simulink library "momentum_flight_control_v1"  (R2022a)
settings: Solver=VariableStepAuto  StartTime=0.0  StopTime=10.0  RelTol=1e-3
undefined symbols (not defined in the file): biasVectorConstraint_feet, Config, ConstraintMatrix_feet, DiscIntNeverNeededParam, Frames
libraries: WBToolboxLibrary x40
(part 1 of 2)
settings Model: Creator=gnava  LastModifiedBy=gnava
settings SolverCC: AlgebraicLoopSolver=TrustRegion
settings DebuggingCC: UnconnectedInputMsg=warning  UnconnectedOutputMsg=warning  UnconnectedLineMsg=warning  SFMachineParentedDataDiag=warning
settings RTWCC: DLArmComputeVersion=19.05

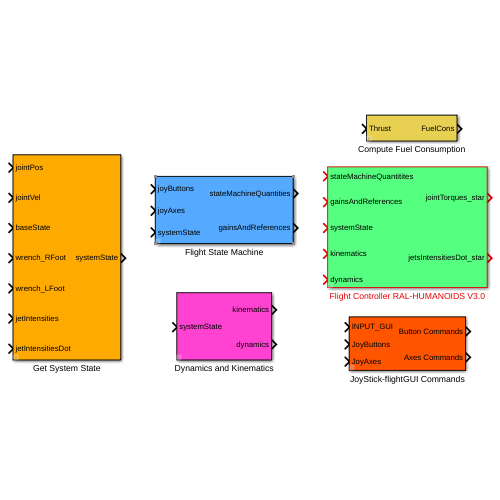
[thumbnail: Simulink's stored preview of the top-level diagram]
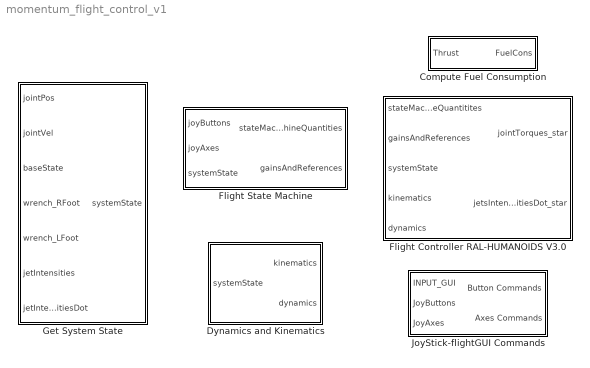
== system momentum_flight_control_v1 ==
  Compute Fuel Consumption : Subsystem  mask{Parameter1=Config}
      mask prompts: Parameter1 "Specify the parameters struct"
      mask DialogControl DescGroupVar Prompt: Compute Fuel Consumption
      mask DialogControl DescTextVar Prompt: Calculates the fuel consumption while flying.
  Dynamics and Kinematics : Subsystem  mask{Parameter1=Config, Parameter2=Frames}
      mask prompts: Parameter1 "Specify the parameters struct"; Parameter2 "Specify the frame names struct"
      mask DialogControl DescGroupVar Prompt: Dynamics and Kinematics
      mask DialogControl DescTextVar Prompt: Computes the dynamics and kinematics quantities that are required by the iRonCub flight controller.
  Flight Controller RAL-HUMANOIDS V3.0 : Subsystem  mask{Parameter1=Config}
      mask prompts: Parameter1 "Specify the parameters struct"
      mask DialogControl DescGroupVar Prompt: Flight Controller RAL-HUMANOIDS
      mask DialogControl DescTextVar Prompt: This block implements the momentum-based flight controller decribed in RAL 2018 and HUMANOIDS 2018 papers.
      mask DialogControl Control3 Prompt: References:
      mask DialogControl Control5 Prompt: RAL 2018 paper
      mask DialogControl Control5 Callback: web https://ieeexplore.ieee.org/document/7997895
      mask DialogControl Control6 Prompt: HUMANOIDS 2018 paper
      mask DialogControl Control6 Callback: web https://ieeexplore.ieee.org/document/8624985
  Flight State Machine : Subsystem  mask{Parameter1=Config, Parameter2=Frames}
      mask prompts: Parameter1 "Specify the parameters struct"; Parameter2 "Specify the frame names struct"
      mask DialogControl DescGroupVar Prompt: Flight State Machine
      mask DialogControl DescTextVar Prompt: Implements a state machine that allows iRonCub to take off, fly, and land. It also allows the user to provide reference trajectories to the robot via joypad or a control GUI.
  Get System State : Subsystem  mask{Parameter1=Frames}
      mask prompts: Parameter1 "Specify the frame names struct"
      mask DialogControl DescGroupVar Prompt: Get System State
      mask DialogControl DescTextVar Prompt: Computes the iRonCub state vector while flying.
      mask DialogControl DescGroupVar_copy Prompt: Parameters
  JoyStick-flightGUI Commands : Subsystem  mask{Parameter1=Config}
      mask prompts: Parameter1 "Specify the parameters struct"
      mask DialogControl DescGroupVar Prompt: Joystick/flightGUI Commands
      mask DialogControl DescTextVar Prompt: Generates commands for the flight state machine. Commands are provided by the user either using a joypad or with the native GUI.

== system momentum_flight_control_v1/Compute Fuel Consumption ==
  Thrust : Inport
  Discrete-Time Integrator : DiscreteIntegrator  SampleTime=Config.tStep  ICPrevOutput=DiscIntNeverNeededParam  ICPrevScaledInput=DiscIntNeverNeededParam
  Get the Current Fuel Consumption : MATLAB Function  TreatAsAtomicUnit=on
  FuelCons : Outport
  wires:
  Thrust/1 -> Get the Current Fuel Consumption/1(thrusts)
  Get the Current Fuel Consumption/1(fuelConsCurr) -> Discrete-Time Integrator/1
  Discrete-Time Integrator/1 -> FuelCons/1

== system momentum_flight_control_v1/Dynamics and Kinematics ==
  systemState : Inport
  Bus Creator1 : BusCreator  Inputs=5
  Bus Creator2 : BusCreator  Inputs=12
  Bus Selector : BusSelector  OutputSignals=w_H_b,jointPos,w_baseTwist,jointVel
  Dynamic Quantities : Subsystem
  Kinematic Quantities : Subsystem
  kinematics : Outport  VectorParamsAs1DForOutWhenUnconnected=off
  dynamics : Outport  Port=2  VectorParamsAs1DForOutWhenUnconnected=off
  wires:
  systemState/1 -> Bus Selector/1
  Bus Selector/1 -> Dynamic Quantities/2(w_H_b), Kinematic Quantities/1(w_H_b)  "<w_H_b>"
  Bus Selector/2 -> Dynamic Quantities/3(jointPos), Kinematic Quantities/2(jointPos)  "<jointPos>"
  Bus Selector/3 -> Dynamic Quantities/4(w_baseTwist), Kinematic Quantities/3(w_baseTwist)  "<w_baseTwist>"
  Bus Selector/4 -> Dynamic Quantities/5(jointVel), Kinematic Quantities/4(jointVel)  "<jointVel>"
  Dynamic Quantities/4(CMM) -> Bus Creator1/4  "CMM"
  Dynamic Quantities/3(L) -> Bus Creator1/3  "L"
  Dynamic Quantities/2("h ") -> Bus Creator1/2  "h"
  Dynamic Quantities/1(M) -> Bus Creator1/1  "M"
  Bus Creator1/1 -> dynamics/1
  Bus Creator2/1 -> kinematics/1
  Kinematic Quantities/1(J_jets) -> Bus Creator2/1  "J_jets"
  Kinematic Quantities/2(J_CoM) -> Bus Creator2/2  "J_CoM"
  Kinematic Quantities/3(w_R_b) -> Bus Creator2/3  "w_R_b"
  Kinematic Quantities/4(J_LFoot) -> Bus Creator2/4  "J_LFoot"
  Kinematic Quantities/5(J_RFoot) -> Bus Creator2/5  "J_RFoot"
  Kinematic Quantities/6(JDot_LFoot_nu) -> Bus Creator2/6  "JDot_LFoot_nu"
  Kinematic Quantities/7(JDot_RFoot_nu) -> Bus Creator2/7  "JDot_RFoot_nu"
  Kinematic Quantities/8(w_H_LFoot) -> Bus Creator2/8  "w_H_LFoot"
  Kinematic Quantities/9(w_H_RFoot) -> Bus Creator2/9  "w_H_RFoot"
  Kinematic Quantities/10(matrixOfJetsAxes) -> Bus Creator2/10  "matrixOfJetAxes"
  Kinematic Quantities/11(matrixOfJetsArms) -> Bus Creator2/11  "matrixOfJetsArms"
  Kinematic Quantities/12(posCoM) -> Bus Creator2/12, Dynamic Quantities/1(posCoM)  "posCoM"
  Dynamic Quantities/5(w_I_c) -> Bus Creator1/5  "w_I_c"

== system momentum_flight_control_v1/Flight Controller RAL-HUMANOIDS V3.0 ==
  stateMachineQuantitites : Inport
  gainsAndReferences : Inport  Port=2
  systemState : Inport  Port=3
  kinematics : Inport  Port=4
  dynamics : Inport  Port=5
  Joint Torque Control for Flying : Subsystem
  Momentum Control for Flying : Subsystem
  jointTorques_star : Outport  VectorParamsAs1DForOutWhenUnconnected=off
  jetsIntensitiesDot_star : Outport  Port=2  VectorParamsAs1DForOutWhenUnconnected=off
  wires:
  stateMachineQuantitites/1 -> Joint Torque Control for Flying/3(stateMachineQuantitites), Momentum Control for Flying/1(stateMachineQuantitites)
  gainsAndReferences/1 -> Joint Torque Control for Flying/4(gainsAndReferences), Momentum Control for Flying/2(gainsAndReferences)
  systemState/1 -> Joint Torque Control for Flying/5(systemState), Momentum Control for Flying/3(systemState)
  kinematics/1 -> Joint Torque Control for Flying/6(kinematics), Momentum Control for Flying/4(kinematics)
  dynamics/1 -> Joint Torque Control for Flying/7(dynamics), Momentum Control for Flying/5(dynamics)
  Momentum Control for Flying/2(contactForces_star) -> Joint Torque Control for Flying/2(contactForces_star)
  Joint Torque Control for Flying/1(jointTorques_star) -> jointTorques_star/1
  Momentum Control for Flying/3(jetsIntensitiesDot_star) -> jetsIntensitiesDot_star/1
  Momentum Control for Flying/1(jointVel_star) -> Joint Torque Control for Flying/1(jointVel_star)

== system momentum_flight_control_v1/Flight State Machine ==
  joyButtons : Inport
  joyAxes : Inport  Port=2
  systemState : Inport  Port=3
  Bus Selector : BusSelector  OutputSignals=jointPos
  Compute Gains And References : Subsystem
  Take Off/Landing State Detector : Subsystem
  stateMachineQuantities : Outport  VectorParamsAs1DForOutWhenUnconnected=off
  gainsAndReferences : Outport  Port=2  VectorParamsAs1DForOutWhenUnconnected=off
  wires:
  systemState/1 -> Take Off/Landing State Detector/1(systemState), Compute Gains And References/3(systemState), Bus Selector/1
  joyButtons/1 -> Take Off/Landing State Detector/2(joyButtons), Compute Gains And References/2(joyButtons)
  joyAxes/1 -> Compute Gains And References/1(joyAxes)
  Compute Gains And References/1(gainsAndReferences) -> gainsAndReferences/1
  Bus Selector/1 -> Compute Gains And References/4(jointPos)  "<jointPos>"
  Take Off/Landing State Detector/1(stateMachineQuantities) -> stateMachineQuantities/1, Compute Gains And References/5(stateMachineQuantities)

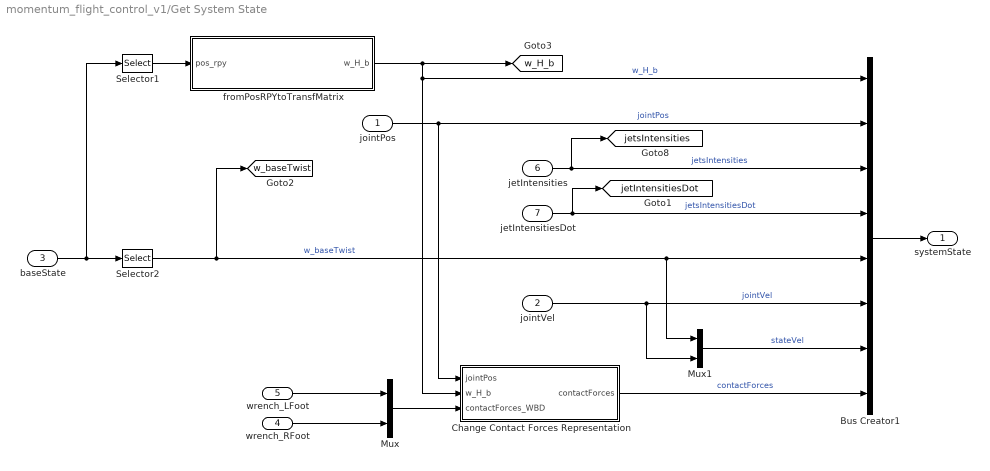
== system momentum_flight_control_v1/Get System State ==
  jointPos : Inport
  jointVel : Inport  Port=2
  baseState : Inport  Port=3
  wrench_RFoot : Inport  Port=4
  wrench_LFoot : Inport  Port=5
  jetIntensities : Inport  Port=6
  jetIntensitiesDot : Inport  Port=7
  Bus Creator1 : BusCreator  Inputs=8
  Change Contact Forces Representation : Subsystem
  Mux : Mux  Inputs=2
  Mux1 : Mux  Inputs=2
  Selector1 : Selector  InputPortWidth=18  IndexOptions=Index vector (dialog)  Indices=[1:6]  OutputSizes=1
  Selector2 : Selector  InputPortWidth=18  IndexOptions=Index vector (dialog)  Indices=[7:12]  OutputSizes=1
  fromPosRPYtoTransfMatrix : MATLAB Function  TreatAsAtomicUnit=on
  systemState : Outport  VectorParamsAs1DForOutWhenUnconnected=off
  tag scope: jetIntensitiesDot=global, jetsIntensities=global, w_H_b=global, w_baseTwist=global
  wires:
  fromPosRPYtoTransfMatrix/1(w_H_b) -> [w_H_b], Change Contact Forces Representation/2(w_H_b), Bus Creator1/1  "w_H_b"
  Mux1/1 -> Bus Creator1/7  "stateVel"
  jetIntensitiesDot/1 -> [jetIntensitiesDot], Bus Creator1/4  "jetsIntensitiesDot"
  wrench_RFoot/1 -> Mux/2
  Mux/1 -> Change Contact Forces Representation/3(contactForces_WBD)
  jointPos/1 -> Change Contact Forces Representation/1(jointPos), Bus Creator1/2  "jointPos"
  jetIntensities/1 -> Bus Creator1/3, [jetsIntensities]  "jetsIntensities"
  Bus Creator1/1 -> systemState/1
  wrench_LFoot/1 -> Mux/1
  Selector1/1 -> fromPosRPYtoTransfMatrix/1(pos_rpy)
  jointVel/1 -> Mux1/2, Bus Creator1/6  "jointVel"
  baseState/1 -> Selector1/1, Selector2/1
  Selector2/1 -> [w_baseTwist], Mux1/1, Bus Creator1/5  "w_baseTwist"
  Change Contact Forces Representation/1(contactForces) -> Bus Creator1/8  "contactForces"

== system momentum_flight_control_v1/JoyStick-flightGUI Commands ==
  INPUT_GUI : Inport
  JoyButtons : Inport  Port=2
  JoyAxes : Inport  Port=3
  Constant : Constant  Value=Config.USE_NATIVE_GUI
  Replace Joystick with Native GUI : MATLAB Function  TreatAsAtomicUnit=on
  Switch1 : Switch  Criteria=u2 > Threshold  SaturateOnIntegerOverflow=off  InputSameDT=off
  Switch2 : Switch  Criteria=u2 > Threshold  SaturateOnIntegerOverflow=off  InputSameDT=off
  Button Commands : Outport  VectorParamsAs1DForOutWhenUnconnected=off
  Axes Commands : Outport  Port=2  VectorParamsAs1DForOutWhenUnconnected=off
  wires:
  INPUT_GUI/1 -> Replace Joystick with Native GUI/1(gui_input)
  Switch1/1 -> Button Commands/1
  Switch2/1 -> Axes Commands/1
  Constant/1 -> Switch2/2, Switch1/2
  JoyButtons/1 -> Switch1/3
  JoyAxes/1 -> Switch2/3
  Replace Joystick with Native GUI/2(joyAxes) -> Switch2/1
  Replace Joystick with Native GUI/1(joyButtons) -> Switch1/1

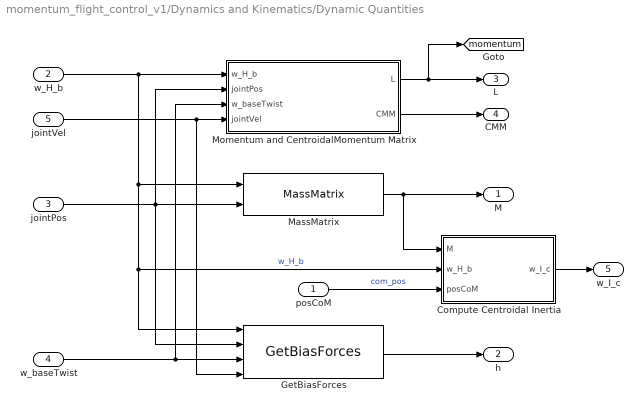
== system momentum_flight_control_v1/Dynamics and Kinematics/Dynamic Quantities ==
  posCoM : Inport
  w_H_b : Inport  Port=2
  jointPos : Inport  Port=3
  w_baseTwist : Inport  Port=4
  jointVel : Inport  Port=5
  Compute Centroidal Inertia : Subsystem
  GetBiasForces : WBToolboxLibrary/Model/Dynamics/GetBiasForces
      settings: SourceProductName=WholeBodyToolbox
  MassMatrix : WBToolboxLibrary/Model/Dynamics/MassMatrix
      settings: SourceProductName=WholeBodyToolbox
  Momentum and CentroidalMomentum Matrix : Subsystem
  M : Outport  VectorParamsAs1DForOutWhenUnconnected=off
  "h " : Outport  Port=2  VectorParamsAs1DForOutWhenUnconnected=off
  L : Outport  Port=3  VectorParamsAs1DForOutWhenUnconnected=off
  CMM : Outport  Port=4  VectorParamsAs1DForOutWhenUnconnected=off
  w_I_c : Outport  Port=5  VectorParamsAs1DForOutWhenUnconnected=off
  tag scope: momentum=global
  wires:
  w_H_b/1 -> Momentum and CentroidalMomentum Matrix/1(w_H_b), GetBiasForces/1, Compute Centroidal Inertia/2(w_H_b), MassMatrix/1  "w_H_b"
  w_baseTwist/1 -> Momentum and CentroidalMomentum Matrix/3(w_baseTwist), GetBiasForces/3
  jointVel/1 -> Momentum and CentroidalMomentum Matrix/4(jointVel), GetBiasForces/4
  MassMatrix/1 -> Compute Centroidal Inertia/1(M), M/1
  GetBiasForces/1 -> "h "/1
  Momentum and CentroidalMomentum Matrix/2(CMM) -> CMM/1
  Momentum and CentroidalMomentum Matrix/1(L) -> L/1, [momentum]
  jointPos/1 -> GetBiasForces/2, MassMatrix/2, Momentum and CentroidalMomentum Matrix/2(jointPos)
  Compute Centroidal Inertia/1(w_I_c) -> w_I_c/1
  posCoM/1 -> Compute Centroidal Inertia/3(posCoM)  "com_pos"

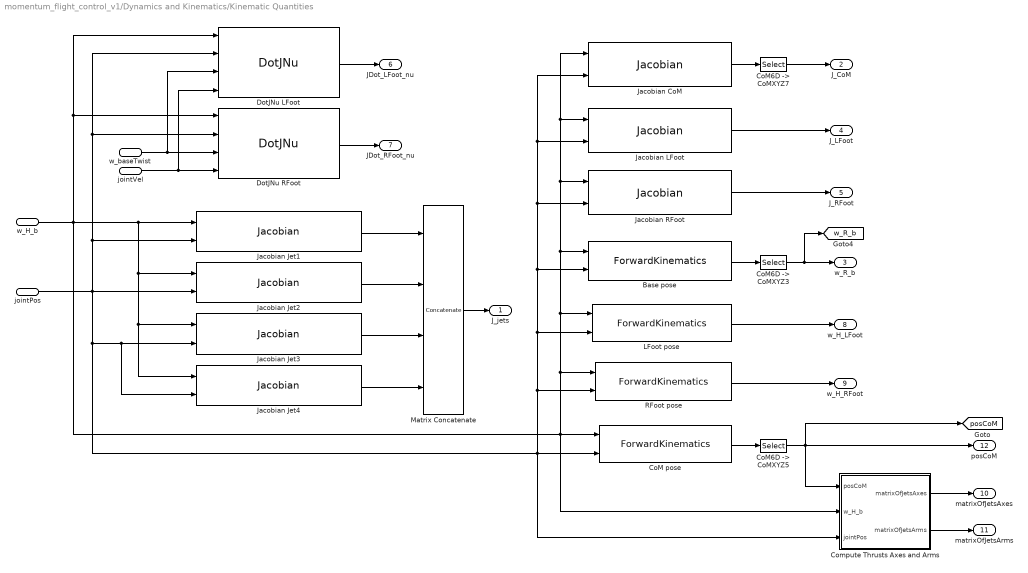
== system momentum_flight_control_v1/Dynamics and Kinematics/Kinematic Quantities ==
  w_H_b : Inport
  jointPos : Inport  Port=2
  w_baseTwist : Inport  Port=3
  jointVel : Inport  Port=4
  Base pose : WBToolboxLibrary/Model/Kinematics/ForwardKinematics  frameName=Frames.BASE_LINK
      settings: SourceProductName=WholeBodyToolbox
  CoM pose : WBToolboxLibrary/Model/Kinematics/ForwardKinematics  frameName=Frames.COM_FRAME
      settings: SourceProductName=WholeBodyToolbox
  "CoM6D -> CoMXYZ3" : Selector  NumberOfDimensions=2  InputPortWidth=7  IndexOptions=Index vector (dialog),Index vector (dialog)  Indices=[1 2 3],[1 2 3]  OutputSizes=1,1
  "CoM6D -> CoMXYZ5" : Selector  NumberOfDimensions=2  InputPortWidth=7  IndexOptions=Index vector (dialog),Index vector (dialog)  Indices=[1 2 3],[4]  OutputSizes=1,1
  "CoM6D -> CoMXYZ7" : Selector  NumberOfDimensions=2  InputPortWidth=7  IndexOptions=Index vector (dialog),Index vector (dialog)  Indices=[1 2 3],[1:6+Config.N_DOF]  OutputSizes=1,1
  Compute Thrusts Axes and Arms : Subsystem
  DotJNu LFoot : WBToolboxLibrary/Model/Jacobians/DotJNu  frameName=Frames.LFOOT_FRAME
      settings: SourceProductName=WholeBodyToolbox
  DotJNu RFoot : WBToolboxLibrary/Model/Jacobians/DotJNu  frameName=Frames.RFOOT_FRAME
      settings: SourceProductName=WholeBodyToolbox
  Jacobian CoM : WBToolboxLibrary/Model/Jacobians/Jacobian  frameName=Frames.COM_FRAME
      settings: SourceProductName=WholeBodyToolbox
  Jacobian Jet1 : WBToolboxLibrary/Model/Jacobians/Jacobian  frameName=Frames.JET1_FRAME
      settings: SourceProductName=WholeBodyToolbox
  Jacobian Jet2 : WBToolboxLibrary/Model/Jacobians/Jacobian  frameName=Frames.JET2_FRAME
      settings: SourceProductName=WholeBodyToolbox
  Jacobian Jet3 : WBToolboxLibrary/Model/Jacobians/Jacobian  frameName=Frames.JET3_FRAME
      settings: SourceProductName=WholeBodyToolbox
  Jacobian Jet4 : WBToolboxLibrary/Model/Jacobians/Jacobian  frameName=Frames.JET4_FRAME
      settings: SourceProductName=WholeBodyToolbox
  Jacobian LFoot : WBToolboxLibrary/Model/Jacobians/Jacobian  frameName=Frames.LFOOT_FRAME
      settings: SourceProductName=WholeBodyToolbox
  Jacobian RFoot : WBToolboxLibrary/Model/Jacobians/Jacobian  frameName=Frames.RFOOT_FRAME
      settings: SourceProductName=WholeBodyToolbox
  LFoot pose : WBToolboxLibrary/Model/Kinematics/ForwardKinematics  frameName=Frames.LFOOT_FRAME
      settings: SourceProductName=WholeBodyToolbox
  Matrix Concatenate : Concatenate  NumInputs=4  Mode=Multidimensional array
  RFoot pose : WBToolboxLibrary/Model/Kinematics/ForwardKinematics  frameName=Frames.RFOOT_FRAME
      settings: SourceProductName=WholeBodyToolbox
  J_jets : Outport  VectorParamsAs1DForOutWhenUnconnected=off
  J_CoM : Outport  Port=2  VectorParamsAs1DForOutWhenUnconnected=off
  w_R_b : Outport  Port=3  VectorParamsAs1DForOutWhenUnconnected=off
  J_LFoot : Outport  Port=4  VectorParamsAs1DForOutWhenUnconnected=off
  J_RFoot : Outport  Port=5  VectorParamsAs1DForOutWhenUnconnected=off
  JDot_LFoot_nu : Outport  Port=6  VectorParamsAs1DForOutWhenUnconnected=off
  JDot_RFoot_nu : Outport  Port=7  VectorParamsAs1DForOutWhenUnconnected=off
  w_H_LFoot : Outport  Port=8  VectorParamsAs1DForOutWhenUnconnected=off
  w_H_RFoot : Outport  Port=9  VectorParamsAs1DForOutWhenUnconnected=off
  matrixOfJetsAxes : Outport  Port=10  VectorParamsAs1DForOutWhenUnconnected=off
  matrixOfJetsArms : Outport  Port=11  VectorParamsAs1DForOutWhenUnconnected=off
  posCoM : Outport  Port=12  VectorParamsAs1DForOutWhenUnconnected=off
  tag scope: posCoM=global, w_R_b=global
  wires:
  Matrix Concatenate/1 -> J_jets/1
  CoM pose/1 -> "CoM6D -> CoMXYZ5"/1
  "CoM6D -> CoMXYZ5"/1 -> posCoM/1, [posCoM], Compute Thrusts Axes and Arms/1(posCoM)
  w_H_b/1 -> LFoot pose/1, Base pose/1, Jacobian LFoot/1, Jacobian CoM/1, Jacobian RFoot/1, RFoot pose/1, CoM pose/1, Compute Thrusts Axes and Arms/2(w_H_b), DotJNu LFoot/1, DotJNu RFoot/1, Jacobian Jet4/1, Jacobian Jet3/1, Jacobian Jet2/1, Jacobian Jet1/1
  "CoM6D -> CoMXYZ3"/1 -> w_R_b/1, [w_R_b]
  jointPos/1 -> Jacobian Jet4/2, Jacobian Jet3/2, Compute Thrusts Axes and Arms/3(jointPos), LFoot pose/2, Jacobian RFoot/2, Jacobian LFoot/2, Jacobian CoM/2, Base pose/2, RFoot pose/2, CoM pose/2, Jacobian Jet2/2, DotJNu LFoot/2, DotJNu RFoot/2, Jacobian Jet1/2
  Jacobian CoM/1 -> "CoM6D -> CoMXYZ7"/1
  Jacobian RFoot/1 -> J_RFoot/1
  Jacobian LFoot/1 -> J_LFoot/1
  DotJNu RFoot/1 -> JDot_RFoot_nu/1
  DotJNu LFoot/1 -> JDot_LFoot_nu/1
  jointVel/1 -> DotJNu RFoot/4, DotJNu LFoot/4
  w_baseTwist/1 -> DotJNu LFoot/3, DotJNu RFoot/3
  RFoot pose/1 -> w_H_RFoot/1
  LFoot pose/1 -> w_H_LFoot/1
  Base pose/1 -> "CoM6D -> CoMXYZ3"/1
  Compute Thrusts Axes and Arms/2(matrixOfJetsArms) -> matrixOfJetsArms/1
  Compute Thrusts Axes and Arms/1(matrixOfJetsAxes) -> matrixOfJetsAxes/1
  Jacobian Jet1/1 -> Matrix Concatenate/1
  Jacobian Jet2/1 -> Matrix Concatenate/2
  Jacobian Jet3/1 -> Matrix Concatenate/3
  Jacobian Jet4/1 -> Matrix Concatenate/4
  "CoM6D -> CoMXYZ7"/1 -> J_CoM/1

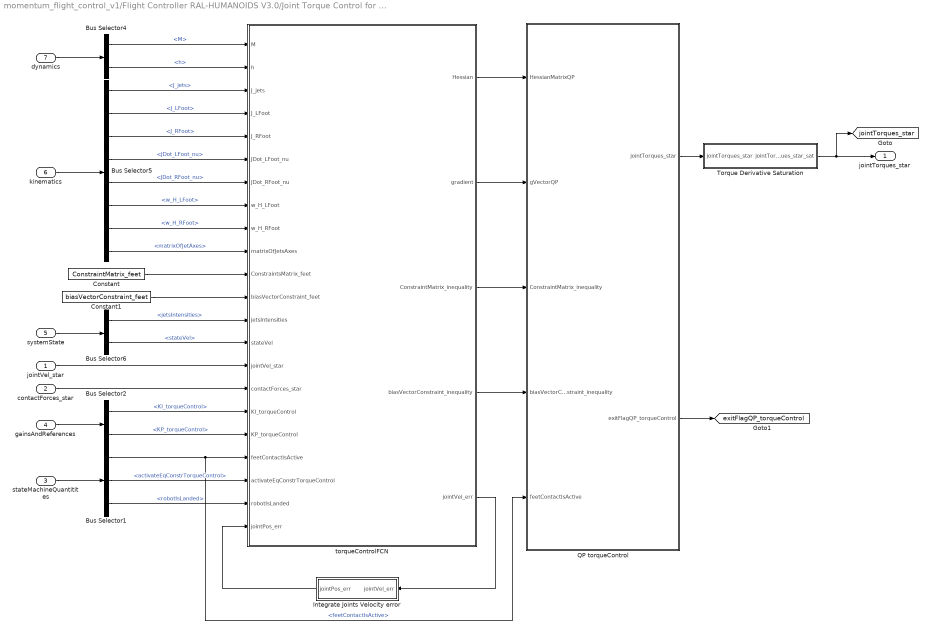
== system momentum_flight_control_v1/Flight Controller RAL-HUMANOIDS V3.0/Joint Torque Control for Flying ==
  jointVel_star : Inport
  contactForces_star : Inport  Port=2
  stateMachineQuantitites : Inport  Port=3
  gainsAndReferences : Inport  Port=4
  systemState : Inport  Port=5
  kinematics : Inport  Port=6
  dynamics : Inport  Port=7
  Bus Selector1 : BusSelector  OutputSignals=feetContactIsActive,activateEqConstrTorqueControl,robotIsLanded
  Bus Selector2 : BusSelector  OutputSignals=KI_torqueControl,KP_torqueControl
  Bus Selector4 : BusSelector  OutputSignals=M,h
  Bus Selector5 : BusSelector  OutputSignals=J_jets,J_LFoot,J_RFoot,JDot_LFoot_nu,JDot_RFoot_nu,w_H_LFoot,w_H_RFoot,matrixOfJetAxes
  Bus Selector6 : BusSelector  OutputSignals=jetsIntensities,stateVel
  Constant : Constant  Value=ConstraintMatrix_feet
  Constant1 : Constant  Value=biasVectorConstraint_feet
  Integrate Joints Velocity error : Subsystem
  QP torqueControl : Subsystem
  Torque Derivative Saturation : Subsystem
  torqueControlFCN : MATLAB Function  TreatAsAtomicUnit=on
  jointTorques_star : Outport  VectorParamsAs1DForOutWhenUnconnected=off
  tag scope: exitFlagQP_torqueControl=global, jointTorques_star=global
  wires:
  Bus Selector6/2 -> torqueControlFCN/14(stateVel)  "<stateVel>"
  dynamics/1 -> Bus Selector4/1
  systemState/1 -> Bus Selector6/1
  kinematics/1 -> Bus Selector5/1
  Bus Selector4/1 -> torqueControlFCN/1(M)  "<M>"
  Bus Selector4/2 -> torqueControlFCN/2(h)  "<h>"
  Bus Selector5/1 -> torqueControlFCN/3(J_jets)  "<J_jets>"
  Bus Selector5/2 -> torqueControlFCN/4(J_LFoot)  "<J_LFoot>"
  Bus Selector5/3 -> torqueControlFCN/5(J_RFoot)  "<J_RFoot>"
  Bus Selector5/4 -> torqueControlFCN/6(JDot_LFoot_nu)  "<JDot_LFoot_nu>"
  Bus Selector5/5 -> torqueControlFCN/7(JDot_RFoot_nu)  "<JDot_RFoot_nu>"
  Bus Selector5/6 -> torqueControlFCN/8(w_H_LFoot)  "<w_H_LFoot>"
  Bus Selector5/7 -> torqueControlFCN/9(w_H_RFoot)  "<w_H_RFoot>"
  Constant1/1 -> torqueControlFCN/12(biasVectorConstraint_feet)
  Constant/1 -> torqueControlFCN/11(ConstraintsMatrix_feet)
  contactForces_star/1 -> torqueControlFCN/16(contactForces_star)
  QP torqueControl/1(jointTorques_star) -> Torque Derivative Saturation/1(jointTorques_star)
  QP torqueControl/2(exitFlagQP_torqueControl) -> [exitFlagQP_torqueControl]
  Bus Selector6/1 -> torqueControlFCN/13(jetsIntensities)  "<jetsIntensities>"
  stateMachineQuantitites/1 -> Bus Selector1/1
  Bus Selector1/1 -> QP torqueControl/5(feetContactIsActive), torqueControlFCN/19(feetContactIsActive)  "<feetContactIsActive>"
  gainsAndReferences/1 -> Bus Selector2/1
  Bus Selector2/1 -> torqueControlFCN/17(KI_torqueControl)  "<KI_torqueControl>"
  Bus Selector2/2 -> torqueControlFCN/18(KP_torqueControl)  "<KP_torqueControl>"
  torqueControlFCN/1(Hessian) -> QP torqueControl/1(HessianMatrixQP)
  torqueControlFCN/2(gradient) -> QP torqueControl/2(gVectorQP)
  torqueControlFCN/3(ConstraintMatrix_inequality) -> QP torqueControl/3(ConstraintMatrix_inequality)
  torqueControlFCN/4(biasVectorConstraint_inequality) -> QP torqueControl/4(biasVectorConstraint_inequality)
  jointVel_star/1 -> torqueControlFCN/15(jointVel_star)
  Bus Selector5/8 -> torqueControlFCN/10(matrixOfJetsAxes)  "<matrixOfJetAxes>"
  Integrate Joints Velocity error/1(jointPos_err) -> torqueControlFCN/22(jointPos_err)
  torqueControlFCN/5(jointVel_err) -> Integrate Joints Velocity error/1(jointVel_err)
  Bus Selector1/3 -> torqueControlFCN/21(robotIsLanded)  "<robotIsLanded>"
  Bus Selector1/2 -> torqueControlFCN/20(activateEqConstrTorqueControl)  "<activateEqConstrTorqueControl>"
  Torque Derivative Saturation/1(jointTorques_star_sat) -> [jointTorques_star], jointTorques_star/1

== system momentum_flight_control_v1/Flight Controller RAL-HUMANOIDS V3.0/Momentum Control for Flying ==
  stateMachineQuantitites : Inport
  gainsAndReferences : Inport  Port=2
  systemState : Inport  Port=3
  kinematics : Inport  Port=4
  dynamics : Inport  Port=5
  Momentum Control : Subsystem
  QP Solver and Integrate Contact Forces Derivative : Subsystem
  jointVel_star : Outport  VectorParamsAs1DForOutWhenUnconnected=off
  contactForces_star : Outport  Port=2  VectorParamsAs1DForOutWhenUnconnected=off
  jetsIntensitiesDot_star : Outport  Port=3  VectorParamsAs1DForOutWhenUnconnected=off
  wires:
  kinematics/1 -> Momentum Control/3(kinematics)
  dynamics/1 -> Momentum Control/4(dynamics)
  gainsAndReferences/1 -> Momentum Control/5(gainsAndReferences)
  stateMachineQuantitites/1 -> Momentum Control/6(stateMachineQuantitites), QP Solver and Integrate Contact Forces Derivative/5(stateMachineQuantities)
  Momentum Control/1(HessianMatrixQP) -> QP Solver and Integrate Contact Forces Derivative/1(HessianMatrixQP)
  Momentum Control/2(gVectorQP) -> QP Solver and Integrate Contact Forces Derivative/2(gVectorQP)
  Momentum Control/3(lowerBoundQP) -> QP Solver and Integrate Contact Forces Derivative/3(lowerBoundQP)
  Momentum Control/4(uppeBoundQP) -> QP Solver and Integrate Contact Forces Derivative/4(upperBoundQP)
  QP Solver and Integrate Contact Forces Derivative/2(jetsIntensitiesDot_star) -> jetsIntensitiesDot_star/1
  QP Solver and Integrate Contact Forces Derivative/1(contactForces_star) -> Momentum Control/1(contactForces_hat), contactForces_star/1  "WARNING! estimated contact forces are assumed to be coincident with contactForces_star"
  QP Solver and Integrate Contact Forces Derivative/3(jointVel_star) -> jointVel_star/1
  systemState/1 -> Momentum Control/2(systemState), QP Solver and Integrate Contact Forces Derivative/6(systemState)

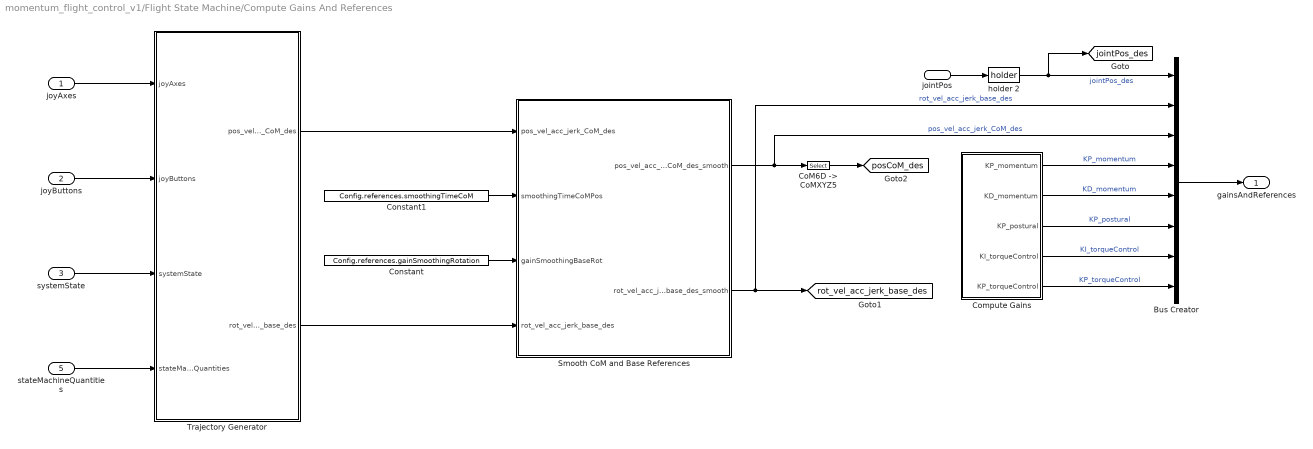
== system momentum_flight_control_v1/Flight State Machine/Compute Gains And References ==
  joyAxes : Inport
  joyButtons : Inport  Port=2
  systemState : Inport  Port=3
  jointPos : Inport  Port=4
  stateMachineQuantities : Inport  Port=5
  Bus Creator : BusCreator  Inputs=8
  "CoM6D -> CoMXYZ5" : Selector  NumberOfDimensions=2  InputPortWidth=7  IndexOptions=Index vector (dialog),Index vector (dialog)  Indices=[1 2 3],[1]  OutputSizes=1,1
  Compute Gains : Subsystem
  Constant : Constant  Value=Config.references.gainSmoothingRotation
  Constant1 : Constant  Value=Config.references.smoothingTimeCoM
  Smooth CoM and Base References : Subsystem
  Trajectory Generator : Subsystem
  holder 2 : WBToolboxLibrary/Utilities/holder 
      settings: SourceProductName=WholeBodyToolbox
  gainsAndReferences : Outport  VectorParamsAs1DForOutWhenUnconnected=off
  tag scope: jointPos_des=global, posCoM_des=global, rot_vel_acc_jerk_base_des=global
  wires:
  "CoM6D -> CoMXYZ5"/1 -> [posCoM_des]
  Smooth CoM and Base References/1(pos_vel_acc_jerk_CoM_des_smooth) -> "CoM6D -> CoMXYZ5"/1, Bus Creator/3  "pos_vel_acc_jerk_CoM_des"
  Constant1/1 -> Smooth CoM and Base References/2(smoothingTimeCoMPos)
  Smooth CoM and Base References/2(rot_vel_acc_jerk_base_des_smooth) -> [rot_vel_acc_jerk_base_des], Bus Creator/2  "rot_vel_acc_jerk_base_des"
  Compute Gains/5(KP_torqueControl) -> Bus Creator/8  "KP_torqueControl"
  Compute Gains/2(KD_momentum) -> Bus Creator/5  "KD_momentum"
  Compute Gains/1(KP_momentum) -> Bus Creator/4  "KP_momentum"
  Compute Gains/3(KP_postural) -> Bus Creator/6  "KP_postural"
  Constant/1 -> Smooth CoM and Base References/3(gainSmoothingBaseRot)
  Bus Creator/1 -> gainsAndReferences/1
  Compute Gains/4(KI_torqueControl) -> Bus Creator/7  "KI_torqueControl"
  holder 2/1 -> Bus Creator/1, [jointPos_des]  "jointPos_des"
  jointPos/1 -> holder 2/1
  joyAxes/1 -> Trajectory Generator/1(joyAxes)
  joyButtons/1 -> Trajectory Generator/2(joyButtons)
  systemState/1 -> Trajectory Generator/3(systemState)
  stateMachineQuantities/1 -> Trajectory Generator/4(stateMachineQuantities)
  Trajectory Generator/1(pos_vel_acc_jerk_CoM_des) -> Smooth CoM and Base References/1(pos_vel_acc_jerk_CoM_des)
  Trajectory Generator/2(rot_vel_acc_jerk_base_des) -> Smooth CoM and Base References/4(rot_vel_acc_jerk_base_des)

== system momentum_flight_control_v1/Flight State Machine/Take Off//Landing State Detector ==
  systemState : Inport
  joyButtons : Inport  Port=2
  Bus Creator : BusCreator  Inputs=6
  Bus Selector : BusSelector  OutputSignals=contactForces
  Demux : Demux  Outputs=[6;6]
  MATLAB Function : MATLAB Function  TreatAsAtomicUnit=on
  Vertical Forces Control : MATLAB Function  TreatAsAtomicUnit=on
  stateMachineQuantities : Outport  VectorParamsAs1DForOutWhenUnconnected=off
  tag scope: stateMachineQuantities=global
  wires:
  Vertical Forces Control/1(decreaseMaxFootVerticalForce) -> Bus Creator/1  "decreaseMaxFootVerticalForce"
  Vertical Forces Control/2(increaseMinFootVerticalForce) -> Bus Creator/2  "increaseMinFootVerticalForce"
  Bus Creator/1 -> [stateMachineQuantities], stateMachineQuantities/1
  systemState/1 -> Bus Selector/1
  joyButtons/1 -> Vertical Forces Control/1(joyButtons)
  Demux/2 -> MATLAB Function/2(wrench_r)
  Demux/1 -> MATLAB Function/1(wrench_l)
  Bus Selector/1 -> Demux/1  "<contactForces>"
  MATLAB Function/1(feetContactIsActive) -> Bus Creator/4  "feetContactIsActive"
  MATLAB Function/2(robotIsLanded) -> Bus Creator/5  "robotIsLanded"
  MATLAB Function/3(oneFootIsInContact) -> Bus Creator/6  "oneFootIsInContact"
  Vertical Forces Control/3(activateEqConstrTorqueControl) -> Bus Creator/3  "activateEqConstrTorqueControl"

== system momentum_flight_control_v1/Get System State/Change Contact Forces Representation ==
  jointPos : Inport
  w_H_b : Inport  Port=2
  contactForces_WBD : Inport  Port=3
  Change Contact Forces Representation : MATLAB Function  TreatAsAtomicUnit=on
  "CoM6D -> CoMXYZ1" : Selector  NumberOfDimensions=2  InputPortWidth=7  IndexOptions=Index vector (dialog),Index vector (dialog)  Indices=[1 2 3],[1 2 3]  OutputSizes=1,1
  "CoM6D -> CoMXYZ3" : Selector  NumberOfDimensions=2  InputPortWidth=7  IndexOptions=Index vector (dialog),Index vector (dialog)  Indices=[1 2 3],[1 2 3]  OutputSizes=1,1
  LFoot Pose : WBToolboxLibrary/Model/Kinematics/ForwardKinematics  frameName=Frames.LFOOT_FRAME
      settings: SourceProductName=WholeBodyToolbox
  Mux : Mux  Inputs=2
  RFoot Pose : WBToolboxLibrary/Model/Kinematics/ForwardKinematics  frameName=Frames.RFOOT_FRAME
      settings: SourceProductName=WholeBodyToolbox
  contactForces : Outport  VectorParamsAs1DForOutWhenUnconnected=off
  tag scope: wrench_LFoot=global, wrench_RFoot=global
  wires:
  Mux/1 -> contactForces/1
  Change Contact Forces Representation/2(mixed_f_r_sole) -> Mux/2, [wrench_RFoot]
  Change Contact Forces Representation/1(mixed_f_l_sole) -> Mux/1, [wrench_LFoot]
  jointPos/1 -> RFoot Pose/2, LFoot Pose/2
  w_H_b/1 -> RFoot Pose/1, LFoot Pose/1
  "CoM6D -> CoMXYZ1"/1 -> Change Contact Forces Representation/2(w_R_l_sole)
  LFoot Pose/1 -> "CoM6D -> CoMXYZ1"/1
  "CoM6D -> CoMXYZ3"/1 -> Change Contact Forces Representation/3(w_R_r_sole)
  RFoot Pose/1 -> "CoM6D -> CoMXYZ3"/1
  contactForces_WBD/1 -> Change Contact Forces Representation/1(contactForces_WBD)

== system momentum_flight_control_v1/Dynamics and Kinematics/Dynamic Quantities/Compute Centroidal Inertia ==
  M : Inport
  w_H_b : Inport  Port=2
  posCoM : Inport  Port=3
  Compute Centroidal Inertia : MATLAB Function  TreatAsAtomicUnit=on
  Selector : Selector  NumberOfDimensions=2  InputPortWidth=3  IndexOptions=Index vector (dialog),Index vector (dialog)  Indices=[1 2 3],4  OutputSizes=1,1
  w_I_c : Outport  VectorParamsAs1DForOutWhenUnconnected=off
  wires:
  M/1 -> Compute Centroidal Inertia/1(M)
  w_H_b/1 -> Selector/1
  Selector/1 -> Compute Centroidal Inertia/3(posBase)
  posCoM/1 -> Compute Centroidal Inertia/2(posCoM)
  Compute Centroidal Inertia/1(w_I_c) -> w_I_c/1

== system momentum_flight_control_v1/Dynamics and Kinematics/Dynamic Quantities/Momentum and CentroidalMomentum Matrix ==
  w_H_b : Inport
  jointPos : Inport  Port=2
  w_baseTwist : Inport  Port=3
  jointVel : Inport  Port=4
  CentroidalMomentum : WBToolboxLibrary/Model/Dynamics/CentroidalMomentum
      settings: SourceProductName=WholeBodyToolbox
  CentroidalTotalMomentumMatrix : WBToolboxLibrary/Model/Jacobians/CentroidalTotalMomentumMatrix
      settings: SourceProductName=WholeBodyToolbox
  L : Outport  VectorParamsAs1DForOutWhenUnconnected=off
  CMM : Outport  Port=2  VectorParamsAs1DForOutWhenUnconnected=off
  wires:
  w_baseTwist/1 -> CentroidalMomentum/3
  CentroidalMomentum/1 -> L/1
  w_H_b/1 -> CentroidalTotalMomentumMatrix/1, CentroidalMomentum/1
  jointPos/1 -> CentroidalTotalMomentumMatrix/2, CentroidalMomentum/2
  jointVel/1 -> CentroidalMomentum/4
  CentroidalTotalMomentumMatrix/1 -> CMM/1

== system momentum_flight_control_v1/Dynamics and Kinematics/Kinematic Quantities/Compute Thrusts Axes and Arms ==
  posCoM : Inport
  w_H_b : Inport  Port=2
  jointPos : Inport  Port=3
  Pose Jet 1 : WBToolboxLibrary/Model/Kinematics/ForwardKinematics  frameName=Frames.JET1_FRAME
      settings: SourceProductName=WholeBodyToolbox
  Pose Jet 2 : WBToolboxLibrary/Model/Kinematics/ForwardKinematics  frameName=Frames.JET2_FRAME
      settings: SourceProductName=WholeBodyToolbox
  Pose Jet 3 : WBToolboxLibrary/Model/Kinematics/ForwardKinematics  frameName=Frames.JET3_FRAME
      settings: SourceProductName=WholeBodyToolbox
  Pose Jet 4 : WBToolboxLibrary/Model/Kinematics/ForwardKinematics  frameName=Frames.JET4_FRAME
      settings: SourceProductName=WholeBodyToolbox
  Thrust Axes and Arms : MATLAB Function  TreatAsAtomicUnit=on
  matrixOfJetsAxes : Outport  VectorParamsAs1DForOutWhenUnconnected=off
  matrixOfJetsArms : Outport  Port=2  VectorParamsAs1DForOutWhenUnconnected=off
  wires:
  Pose Jet 2/1 -> Thrust Axes and Arms/2(w_H_J2)
  jointPos/1 -> Pose Jet 1/2, Pose Jet 2/2, Pose Jet 3/2, Pose Jet 4/2
  Pose Jet 1/1 -> Thrust Axes and Arms/1(w_H_J1)
  Pose Jet 3/1 -> Thrust Axes and Arms/3(w_H_J3)
  Pose Jet 4/1 -> Thrust Axes and Arms/4(w_H_J4)
  Thrust Axes and Arms/1(matrixOfJetsAxes) -> matrixOfJetsAxes/1
  Thrust Axes and Arms/2(matrixOfJetsArms) -> matrixOfJetsArms/1
  w_H_b/1 -> Pose Jet 4/1, Pose Jet 3/1, Pose Jet 2/1, Pose Jet 1/1
  posCoM/1 -> Thrust Axes and Arms/5(posCoM)

== system momentum_flight_control_v1/Flight Controller RAL-HUMANOIDS V3.0/Joint Torque Control for Flying/Integrate Joints Velocity error ==
  jointVel_err : Inport
  Constant : Constant  Value=zeros(Config.N_DOF,1)
  Discrete-Time Integrator1 : DiscreteIntegrator  InitialConditionSource=external  InitialCondition=zeros(Config.N_DOF,1)  SampleTime=Config.tStep  ICPrevOutput=DiscIntNeverNeededParam  ICPrevScaledInput=DiscIntNeverNeededParam
  jointPos_err : Outport  VectorParamsAs1DForOutWhenUnconnected=off
  tag scope: jointPos_err_integral=global
  wires:
  Discrete-Time Integrator1/1 -> jointPos_err/1, [jointPos_err_integral]
  jointVel_err/1 -> Discrete-Time Integrator1/1
  Constant/1 -> Discrete-Time Integrator1/2

== system momentum_flight_control_v1/Flight Controller RAL-HUMANOIDS V3.0/Joint Torque Control for Flying/QP torqueControl ==
  HessianMatrixQP : Inport
  gVectorQP : Inport  Port=2
  ConstraintMatrix_inequality : Inport  Port=3
  biasVectorConstraint_inequality : Inport  Port=4
  feetContactIsActive : Inport  Port=5
  Constant2 : Constant  Value=Config.sat.jointTorquesSaturation
  NOT : Logic  Operator=NOT  IconShape=distinctive  AllPortsSameDT=off  OutDataTypeStr=boolean
  Process QP Inputs Torque Control : MATLAB Function  TreatAsAtomicUnit=on
  QP torqueControl - balancing : Subsystem  TreatAsAtomicUnit=on
  QP torqueControl - flight : Subsystem  TreatAsAtomicUnit=on
  Select QP torqueControl Output : Subsystem
  jointTorques_star : Outport  VectorParamsAs1DForOutWhenUnconnected=off
  exitFlagQP_torqueControl : Outport  Port=2  VectorParamsAs1DForOutWhenUnconnected=off
  wires:
  feetContactIsActive/1 -> Select QP torqueControl Output/3(feetContactIsActive), QP torqueControl - balancing/Enable, NOT/1
  NOT/1 -> QP torqueControl - flight/Enable
  biasVectorConstraint_inequality/1 -> Process QP Inputs Torque Control/4(biasVectorInequalityConstr)
  ConstraintMatrix_inequality/1 -> Process QP Inputs Torque Control/3(InequalityConstrMatrix)
  HessianMatrixQP/1 -> Process QP Inputs Torque Control/1(HessianMatrixQP)
  gVectorQP/1 -> Process QP Inputs Torque Control/2(gVectorQP)
  Constant2/1 -> Process QP Inputs Torque Control/5(jointTorquesSaturation)
  Process QP Inputs Torque Control/8(H_flight) -> QP torqueControl - flight/1(H)
  Process QP Inputs Torque Control/9(g_flight) -> QP torqueControl - flight/2(g)
  Process QP Inputs Torque Control/10(ub_flight) -> QP torqueControl - flight/3(ub)
  Process QP Inputs Torque Control/11(lb_flight) -> QP torqueControl - flight/4(lb)
  Process QP Inputs Torque Control/7(ubEq_balancing) -> QP torqueControl - balancing/7(ubEq)
  Process QP Inputs Torque Control/6(lbEq_balancing) -> QP torqueControl - balancing/6(lbEq)
  Process QP Inputs Torque Control/5(Aeq_balancing) -> QP torqueControl - balancing/5(AEq)
  Process QP Inputs Torque Control/4(lb_balancing) -> QP torqueControl - balancing/4(lb)
  Process QP Inputs Torque Control/3(ub_balancing) -> QP torqueControl - balancing/3(ub)
  Process QP Inputs Torque Control/2(g_balancing) -> QP torqueControl - balancing/2(g)
  Process QP Inputs Torque Control/1(H_balancing) -> QP torqueControl - balancing/1(H)
  QP torqueControl - balancing/1(QPStatus_balancing) -> Select QP torqueControl Output/1(QPStatus_balancing)
  QP torqueControl - balancing/2(QPOutput_balancing) -> Select QP torqueControl Output/2(QPOutput_balancing)
  QP torqueControl - flight/2(QPOutput_flight) -> Select QP torqueControl Output/5(QPOutput_flight)
  QP torqueControl - flight/1(QPStatus_flight) -> Select QP torqueControl Output/4(QPStatus_flight)
  Select QP torqueControl Output/2(exitFlagQP_torqueControl) -> exitFlagQP_torqueControl/1
  Select QP torqueControl Output/1(jointTorques_star) -> jointTorques_star/1

== system momentum_flight_control_v1/Flight Controller RAL-HUMANOIDS V3.0/Joint Torque Control for Flying/Torque Derivative Saturation ==
  jointTorques_star : Inport
  Constant1 : Constant  Value=Config.tStep
  Constant2 : Constant  Value=Config.sat.jointTorquesDotMax
  Saturate Torque Derivative : MATLAB Function  TreatAsAtomicUnit=on
  "holder " : WBToolboxLibrary/Utilities/holder 
      settings: SourceProductName=WholeBodyToolbox
  jointTorques_star_sat : Outport  VectorParamsAs1DForOutWhenUnconnected=off
  wires:
  jointTorques_star/1 -> "holder "/1, Saturate Torque Derivative/1(u)
  Saturate Torque Derivative/1(uSat) -> jointTorques_star_sat/1
  "holder "/1 -> Saturate Torque Derivative/2(u_0)
  Constant1/1 -> Saturate Torque Derivative/3(tStep)
  Constant2/1 -> Saturate Torque Derivative/4(uDotMax)

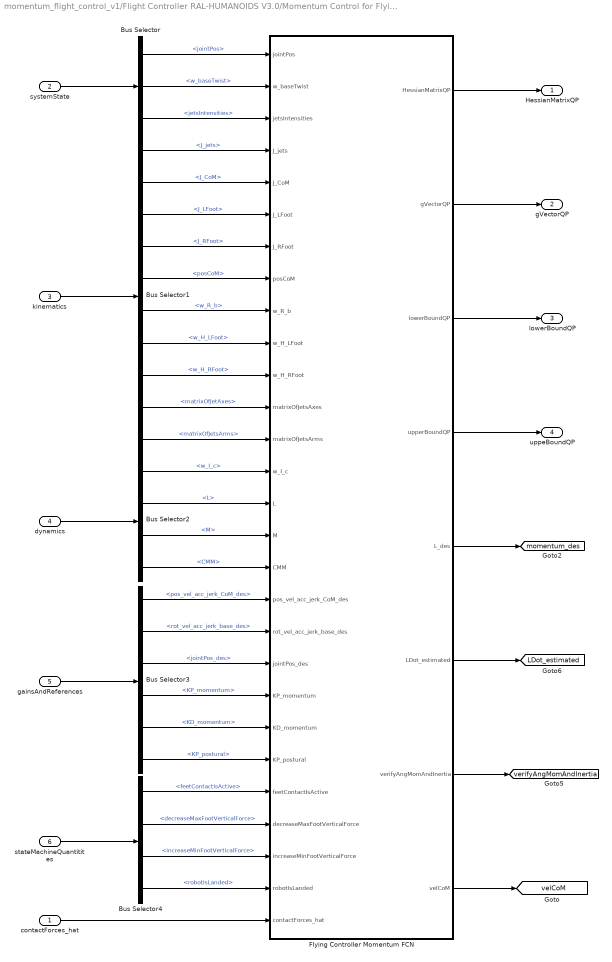
== system momentum_flight_control_v1/Flight Controller RAL-HUMANOIDS V3.0/Momentum Control for Flying/Momentum Control ==
  contactForces_hat : Inport
  systemState : Inport  Port=2
  kinematics : Inport  Port=3
  dynamics : Inport  Port=4
  gainsAndReferences : Inport  Port=5
  stateMachineQuantitites : Inport  Port=6
  Bus Selector : BusSelector  OutputSignals=jointPos,w_baseTwist,jetsIntensities
  Bus Selector1 : BusSelector  OutputSignals=J_jets,J_CoM,J_LFoot,J_RFoot,posCoM,w_R_b,w_H_LFoot,w_H_RFoot,matrixOfJetAxes,matrixOfJetsArms
  Bus Selector2 : BusSelector  OutputSignals=w_I_c,L,M,CMM
  Bus Selector3 : BusSelector  OutputSignals=pos_vel_acc_jerk_CoM_des,rot_vel_acc_jerk_base_des,jointPos_des,KP_momentum,KD_momentum,KP_postural
  Bus Selector4 : BusSelector  OutputSignals=feetContactIsActive,decreaseMaxFootVerticalForce,increaseMinFootVerticalForce,robotIsLanded
  "Flying Controller Momentum FCN " : MATLAB Function  TreatAsAtomicUnit=on
  HessianMatrixQP : Outport  VectorParamsAs1DForOutWhenUnconnected=off
  gVectorQP : Outport  Port=2  VectorParamsAs1DForOutWhenUnconnected=off
  lowerBoundQP : Outport  Port=3  VectorParamsAs1DForOutWhenUnconnected=off
  uppeBoundQP : Outport  Port=4  VectorParamsAs1DForOutWhenUnconnected=off
  tag scope: LDot_estimated=global, momentum_des=global, velCoM=global, verifyAngMomAndInertia=global
  wires:
  systemState/1 -> Bus Selector/1
  Bus Selector3/3 -> "Flying Controller Momentum FCN "/20(jointPos_des)  "<jointPos_des>"
  Bus Selector1/3 -> "Flying Controller Momentum FCN "/6(J_LFoot)  "<J_LFoot>"
  kinematics/1 -> Bus Selector1/1
  Bus Selector/1 -> "Flying Controller Momentum FCN "/1(jointPos)  "<jointPos>"
  Bus Selector1/1 -> "Flying Controller Momentum FCN "/4(J_jets)  "<J_jets>"
  Bus Selector/2 -> "Flying Controller Momentum FCN "/2(w_baseTwist)  "<w_baseTwist>"
  "Flying Controller Momentum FCN "/1(HessianMatrixQP) -> HessianMatrixQP/1
  "Flying Controller Momentum FCN "/4(upperBoundQP) -> uppeBoundQP/1
  "Flying Controller Momentum FCN "/2(gVectorQP) -> gVectorQP/1
  Bus Selector4/1 -> "Flying Controller Momentum FCN "/24(feetContactIsActive)  "<feetContactIsActive>"
  "Flying Controller Momentum FCN "/7(verifyAngMomAndInertia) -> [verifyAngMomAndInertia]
  stateMachineQuantitites/1 -> Bus Selector4/1
  "Flying Controller Momentum FCN "/3(lowerBoundQP) -> lowerBoundQP/1
  Bus Selector3/4 -> "Flying Controller Momentum FCN "/21(KP_momentum)  "<KP_momentum>"
  dynamics/1 -> Bus Selector2/1
  Bus Selector1/2 -> "Flying Controller Momentum FCN "/5(J_CoM)  "<J_CoM>"
  gainsAndReferences/1 -> Bus Selector3/1
  Bus Selector/3 -> "Flying Controller Momentum FCN "/3(jetsIntensities)  "<jetsIntensities>"
  Bus Selector1/4 -> "Flying Controller Momentum FCN "/7(J_RFoot)  "<J_RFoot>"
  Bus Selector1/8 -> "Flying Controller Momentum FCN "/11(w_H_RFoot)  "<w_H_RFoot>"
  Bus Selector2/4 -> "Flying Controller Momentum FCN "/17(CMM)  "<CMM>"
  Bus Selector2/3 -> "Flying Controller Momentum FCN "/16(M)  "<M>"
  "Flying Controller Momentum FCN "/6(LDot_estimated) -> [LDot_estimated]
  Bus Selector3/5 -> "Flying Controller Momentum FCN "/22(KD_momentum)  "<KD_momentum>"
  Bus Selector1/7 -> "Flying Controller Momentum FCN "/10(w_H_LFoot)  "<w_H_LFoot>"
  Bus Selector2/2 -> "Flying Controller Momentum FCN "/15(L)  "<L>"
  Bus Selector3/6 -> "Flying Controller Momentum FCN "/23(KP_postural)  "<KP_postural>"
  "Flying Controller Momentum FCN "/5(L_des) -> [momentum_des]
  Bus Selector1/5 -> "Flying Controller Momentum FCN "/8(posCoM)  "<posCoM>"
  Bus Selector3/2 -> "Flying Controller Momentum FCN "/19(rot_vel_acc_jerk_base_des)  "<rot_vel_acc_jerk_base_des>"
  Bus Selector1/6 -> "Flying Controller Momentum FCN "/9(w_R_b)  "<w_R_b>"
  Bus Selector3/1 -> "Flying Controller Momentum FCN "/18(pos_vel_acc_jerk_CoM_des)  "<pos_vel_acc_jerk_CoM_des>"
  Bus Selector1/9 -> "Flying Controller Momentum FCN "/12(matrixOfJetsAxes)  "<matrixOfJetAxes>"
  Bus Selector1/10 -> "Flying Controller Momentum FCN "/13(matrixOfJetsArms)  "<matrixOfJetsArms>"
  Bus Selector2/1 -> "Flying Controller Momentum FCN "/14(w_I_c)  "<w_I_c>"
  Bus Selector4/2 -> "Flying Controller Momentum FCN "/25(decreaseMaxFootVerticalForce)  "<decreaseMaxFootVerticalForce>"
  Bus Selector4/3 -> "Flying Controller Momentum FCN "/26(increaseMinFootVerticalForce)  "<increaseMinFootVerticalForce>"
  Bus Selector4/4 -> "Flying Controller Momentum FCN "/27(robotIsLanded)  "<robotIsLanded>"
  contactForces_hat/1 -> "Flying Controller Momentum FCN "/28(contactForces_hat)
  "Flying Controller Momentum FCN "/8(velCoM) -> [velCoM]

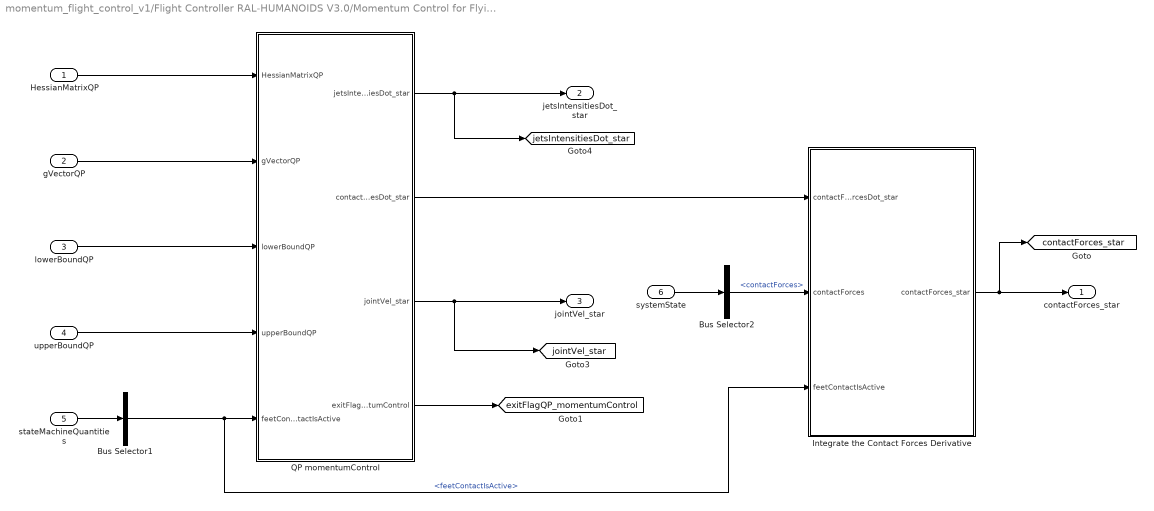
== system momentum_flight_control_v1/Flight Controller RAL-HUMANOIDS V3.0/Momentum Control for Flying/QP Solver and Integrate Contact Forces Derivative ==
  HessianMatrixQP : Inport
  gVectorQP : Inport  Port=2
  lowerBoundQP : Inport  Port=3
  upperBoundQP : Inport  Port=4
  stateMachineQuantities : Inport  Port=5
  systemState : Inport  Port=6
  Bus Selector1 : BusSelector  OutputSignals=feetContactIsActive
  Bus Selector2 : BusSelector  OutputSignals=contactForces
  Integrate the Contact Forces Derivative : Subsystem
  QP momentumControl : Subsystem
  contactForces_star : Outport  VectorParamsAs1DForOutWhenUnconnected=off
  jetsIntensitiesDot_star : Outport  Port=2  VectorParamsAs1DForOutWhenUnconnected=off
  jointVel_star : Outport  Port=3  VectorParamsAs1DForOutWhenUnconnected=off
  tag scope: contactForces_star=global, exitFlagQP_momentumControl=global, jetsIntensitiesDot_star=global, jointVel_star=global
  wires:
  Integrate the Contact Forces Derivative/1(contactForces_star) -> [contactForces_star], contactForces_star/1
  QP momentumControl/2(contactForcesDot_star) -> Integrate the Contact Forces Derivative/1(contactForcesDot_star)
  lowerBoundQP/1 -> QP momentumControl/3(lowerBoundQP)
  upperBoundQP/1 -> QP momentumControl/4(upperBoundQP)
  QP momentumControl/4(exitFlagQP_momentumControl) -> [exitFlagQP_momentumControl]
  gVectorQP/1 -> QP momentumControl/2(gVectorQP)
  stateMachineQuantities/1 -> Bus Selector1/1
  HessianMatrixQP/1 -> QP momentumControl/1(HessianMatrixQP)
  QP momentumControl/1(jetsIntensitiesDot_star) -> jetsIntensitiesDot_star/1, [jetsIntensitiesDot_star]
  QP momentumControl/3(jointVel_star) -> [jointVel_star], jointVel_star/1
  Bus Selector1/1 -> QP momentumControl/5(feetContactIsActive), Integrate the Contact Forces Derivative/3(feetContactIsActive)  "<feetContactIsActive>"
  Bus Selector2/1 -> Integrate the Contact Forces Derivative/2(contactForces)  "<contactForces>"
  systemState/1 -> Bus Selector2/1

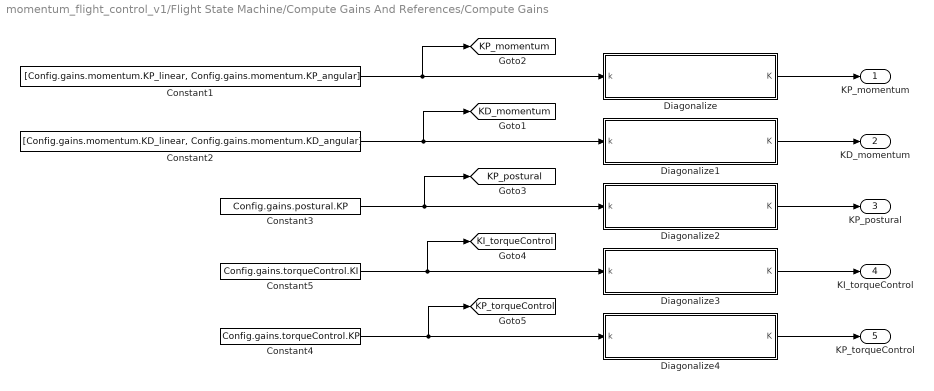
== system momentum_flight_control_v1/Flight State Machine/Compute Gains And References/Compute Gains ==
  Constant1 : Constant  Value=[Config.gains.momentum.KP_linear, Config.gains.momentum.KP_angular]
  Constant2 : Constant  Value=[Config.gains.momentum.KD_linear, Config.gains.momentum.KD_angular]
  Constant3 : Constant  Value=Config.gains.postural.KP
  Constant4 : Constant  Value=Config.gains.torqueControl.KP
  Constant5 : Constant  Value=Config.gains.torqueControl.KI
  Diagonalize : MATLAB Function  TreatAsAtomicUnit=on
  Diagonalize1 : MATLAB Function  TreatAsAtomicUnit=on
  Diagonalize2 : MATLAB Function  TreatAsAtomicUnit=on
  Diagonalize3 : MATLAB Function  TreatAsAtomicUnit=on
  Diagonalize4 : MATLAB Function  TreatAsAtomicUnit=on
  KP_momentum : Outport  VectorParamsAs1DForOutWhenUnconnected=off
  KD_momentum : Outport  Port=2  VectorParamsAs1DForOutWhenUnconnected=off
  KP_postural : Outport  Port=3  VectorParamsAs1DForOutWhenUnconnected=off
  KI_torqueControl : Outport  Port=4  VectorParamsAs1DForOutWhenUnconnected=off
  KP_torqueControl : Outport  Port=5  VectorParamsAs1DForOutWhenUnconnected=off
  tag scope: KD_momentum=global, KI_torqueControl=global, KP_momentum=global, KP_postural=global, KP_torqueControl=global
  wires:
  Diagonalize/1(K) -> KP_momentum/1
  Diagonalize1/1(K) -> KD_momentum/1
  Diagonalize2/1(K) -> KP_postural/1
  Diagonalize3/1(K) -> KI_torqueControl/1
  Diagonalize4/1(K) -> KP_torqueControl/1
  Constant1/1 -> [KP_momentum], Diagonalize/1(k)
  Constant2/1 -> [KD_momentum], Diagonalize1/1(k)
  Constant3/1 -> [KP_postural], Diagonalize2/1(k)
  Constant5/1 -> [KI_torqueControl], Diagonalize3/1(k)
  Constant4/1 -> [KP_torqueControl], Diagonalize4/1(k)

== system momentum_flight_control_v1/Flight State Machine/Compute Gains And References/Smooth CoM and Base References ==
  pos_vel_acc_jerk_CoM_des : Inport
  smoothingTimeCoMPos : Inport  Port=2
  gainSmoothingBaseRot : Inport  Port=3
  rot_vel_acc_jerk_base_des : Inport  Port=4
  Constant : Constant  Value=Config.references.SMOOTH_BASE_ROT_REFERENCES
  Constant1 : Constant  Value=Config.references.SMOOTH_COM_POS_REFERENCES
  Smooth Position References : Subsystem
  Smooth Reference Orientations : Subsystem
  Switch : Switch  Criteria=u2 > Threshold  SaturateOnIntegerOverflow=off  InputSameDT=off
  Switch2 : Switch  Criteria=u2 > Threshold  SaturateOnIntegerOverflow=off  InputSameDT=off
  pos_vel_acc_jerk_CoM_des_smooth : Outport  VectorParamsAs1DForOutWhenUnconnected=off
  rot_vel_acc_jerk_base_des_smooth : Outport  Port=2  VectorParamsAs1DForOutWhenUnconnected=off
  wires:
  Smooth Position References/1(pos_vel_acc_jerk_CoM_des_smooth) -> Switch/1
  smoothingTimeCoMPos/1 -> Smooth Position References/1(smoothingTimeCoMPos)
  pos_vel_acc_jerk_CoM_des/1 -> Switch/3, Smooth Position References/2(pos_vel_acc_jerk_CoM_des)
  Switch2/1 -> rot_vel_acc_jerk_base_des_smooth/1
  Switch/1 -> pos_vel_acc_jerk_CoM_des_smooth/1
  Constant1/1 -> Switch/2
  rot_vel_acc_jerk_base_des/1 -> Smooth Reference Orientations/1(rot_vel_acc_jerk_base_des)
  gainSmoothingBaseRot/1 -> Switch2/3, Smooth Reference Orientations/2(gainSmoothingBaseRot)
  Smooth Reference Orientations/1(rot_acc_vel_jerk_base_des_smooth) -> Switch2/1
  Constant/1 -> Switch2/2

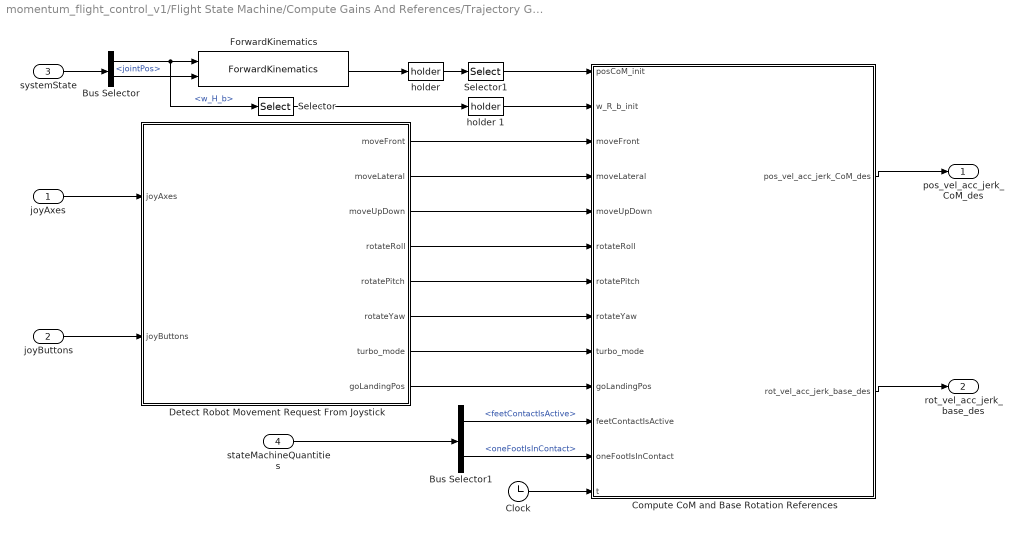
== system momentum_flight_control_v1/Flight State Machine/Compute Gains And References/Trajectory Generator ==
  joyAxes : Inport
  joyButtons : Inport  Port=2
  systemState : Inport  Port=3
  stateMachineQuantities : Inport  Port=4
  Bus Selector : BusSelector  OutputSignals=w_H_b,jointPos
  Bus Selector1 : BusSelector  OutputSignals=feetContactIsActive,oneFootIsInContact
  Clock : Clock
  Compute CoM and Base Rotation References : MATLAB Function  TreatAsAtomicUnit=on
  Detect Robot Movement Request From Joystick : MATLAB Function  TreatAsAtomicUnit=on
  ForwardKinematics : WBToolboxLibrary/Model/Kinematics/ForwardKinematics  frameName=Frames.COM_FRAME
      settings: SourceProductName=WholeBodyToolbox
  Selector : Selector  NumberOfDimensions=2  InputPortWidth=3  IndexOptions=Index vector (dialog),Index vector (dialog)  Indices=[1 2 3],[1 2 3]  OutputSizes=1,1
  Selector1 : Selector  NumberOfDimensions=2  InputPortWidth=3  IndexOptions=Index vector (dialog),Index vector (dialog)  Indices=[1 2 3],[4]  OutputSizes=1,1
  "holder " : WBToolboxLibrary/Utilities/holder 
      settings: SourceProductName=WholeBodyToolbox
  holder 1 : WBToolboxLibrary/Utilities/holder 
      settings: SourceProductName=WholeBodyToolbox
  pos_vel_acc_jerk_CoM_des : Outport  VectorParamsAs1DForOutWhenUnconnected=off
  rot_vel_acc_jerk_base_des : Outport  Port=2  VectorParamsAs1DForOutWhenUnconnected=off
  wires:
  Bus Selector1/2 -> Compute CoM and Base Rotation References/12(oneFootIsInContact)  "<oneFootIsInContact>"
  Detect Robot Movement Request From Joystick/8(goLandingPos) -> Compute CoM and Base Rotation References/10(goLandingPos)
  Selector1/1 -> Compute CoM and Base Rotation References/1(posCoM_init)
  Compute CoM and Base Rotation References/2(rot_vel_acc_jerk_base_des) -> rot_vel_acc_jerk_base_des/1
  joyButtons/1 -> Detect Robot Movement Request From Joystick/2(joyButtons)
  joyAxes/1 -> Detect Robot Movement Request From Joystick/1(joyAxes)
  systemState/1 -> Bus Selector/1
  Clock/1 -> Compute CoM and Base Rotation References/13(t)
  Detect Robot Movement Request From Joystick/6(rotateYaw) -> Compute CoM and Base Rotation References/8(rotateYaw)
  Compute CoM and Base Rotation References/1(pos_vel_acc_jerk_CoM_des) -> pos_vel_acc_jerk_CoM_des/1
  Detect Robot Movement Request From Joystick/4(rotateRoll) -> Compute CoM and Base Rotation References/6(rotateRoll)
  ForwardKinematics/1 -> "holder "/1
  holder 1/1 -> Compute CoM and Base Rotation References/2(w_R_b_init)
  Bus Selector/1 -> Selector/1, ForwardKinematics/1  "<w_H_b>"
  Selector/1 -> holder 1/1
  Bus Selector1/1 -> Compute CoM and Base Rotation References/11(feetContactIsActive)  "<feetContactIsActive>"
  Detect Robot Movement Request From Joystick/5(rotatePitch) -> Compute CoM and Base Rotation References/7(rotatePitch)
  stateMachineQuantities/1 -> Bus Selector1/1
  Detect Robot Movement Request From Joystick/2(moveLateral) -> Compute CoM and Base Rotation References/4(moveLateral)
  Detect Robot Movement Request From Joystick/3(moveUpDown) -> Compute CoM and Base Rotation References/5(moveUpDown)
  Bus Selector/2 -> ForwardKinematics/2  "<jointPos>"
  "holder "/1 -> Selector1/1
  Detect Robot Movement Request From Joystick/1(moveFront) -> Compute CoM and Base Rotation References/3(moveFront)
  Detect Robot Movement Request From Joystick/7(turbo_mode) -> Compute CoM and Base Rotation References/9(turbo_mode)
